simulink library "fsw_bus"  (R2018b)
settings: Solver=VariableStepAuto  StartTime=0.0  StopTime=10.0  RelTol=1e-3
undefined symbols (not defined in the file): fswParams
settings Model: Creator=colem  LastModifiedBy=colem

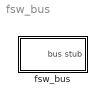
== system fsw_bus ==
  fsw_bus : Subsystem

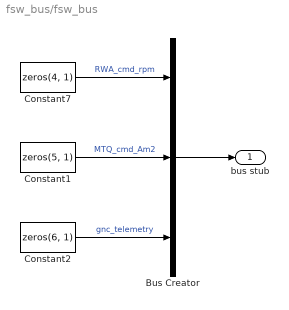
== system fsw_bus/fsw_bus ==
  Bus Creator : BusCreator  Inputs=3
  Constant1 : Constant  Value=zeros(5, 1)  SampleTime=fswParams.sample_time_s
  Constant2 : Constant  Value=zeros(6, 1)  SampleTime=fswParams.sample_time_s
  Constant7 : Constant  Value=zeros(4, 1)  SampleTime=fswParams.sample_time_s
  bus stub : Outport
  wires:
  Constant7/1 -> Bus Creator/1  "RWA_cmd_rpm"
  Bus Creator/1 -> bus stub/1
  Constant1/1 -> Bus Creator/2  "MTQ_cmd_Am2"
  Constant2/1 -> Bus Creator/3  "gnc_telemetry"
